simulink model "Mechanical_module"  (R2023b)
settings: Solver=VariableStepAuto  StartTime=0.0  StopTime=10.0  RelTol=1e-3
undefined symbols (not defined in the file): c_drt, H_gen, H_WTR, k_drt
settings Model: Creator=s183702  LastModifiedBy=s183702

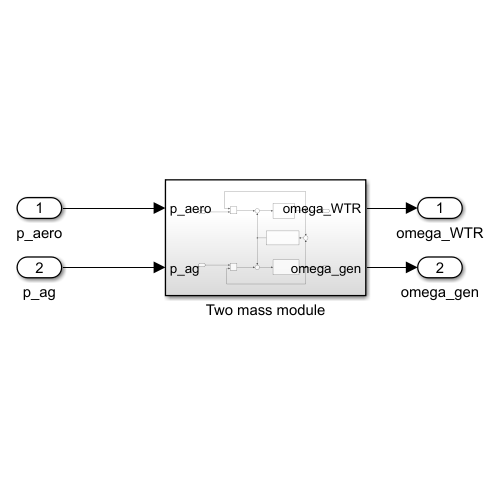
[thumbnail: Simulink's stored preview of the top-level diagram]
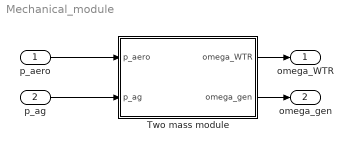
== system Mechanical_module ==
  p_aero : Inport
  p_ag : Inport  Port=2
  Two mass module : Subsystem
  omega_WTR : Outport
  omega_gen : Outport  Port=2
  wires:
  p_ag/1 -> Two mass module/2(p_ag)
  p_aero/1 -> Two mass module/1(p_aero)
  Two mass module/1(omega_WTR) -> omega_WTR/1
  Two mass module/2(omega_gen) -> omega_gen/1

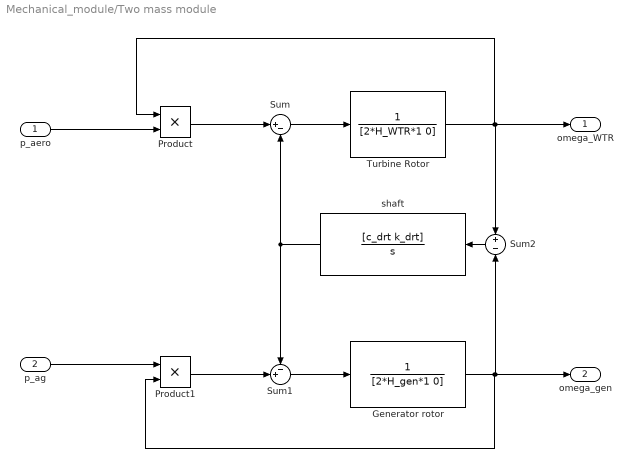
== system Mechanical_module/Two mass module ==
  p_aero : Inport
  p_ag : Inport  Port=2
  Generator rotor : TransferFcn  Denominator=[2*H_gen*1 0]
  Product : Product
  Product1 : Product
  Sum : Sum  Inputs=|+-
  Sum1 : Sum  Inputs=-+|
  Sum2 : Sum  Inputs=+|-
  Turbine Rotor : TransferFcn  Denominator=[2*H_WTR*1 0]
  shaft : TransferFcn  Numerator=[c_drt k_drt]  Denominator=[1 0]
  omega_WTR : Outport
  omega_gen : Outport  Port=2
  wires:
  Product1/1 -> Sum1/2
  Generator rotor/1 -> omega_gen/1, Sum2/2, Product1/2
  shaft/1 -> Sum1/1, Sum/2
  Turbine Rotor/1 -> omega_WTR/1, Sum2/1, Product/1
  Sum/1 -> Turbine Rotor/1
  Sum2/1 -> shaft/1
  p_ag/1 -> Product1/1
  p_aero/1 -> Product/2
  Sum1/1 -> Generator rotor/1
  Product/1 -> Sum/1
